simulink model "OMSv1_1_SSI"  (Simulink 6.5)
settings: Solver=ode4  SolverMode=SingleTasking  StartTime=0.0  StopTime=2.5  FixedStep=0.001  MaxStep=0.001  RelTol=1e-3  AbsTol=1e-3
undefined symbols (not defined in the file): alexlaw, bs_onoff, bs_scale, bsfsacrit, bsfsvcrit, cnsgain, fs_onoff, fs_scale, fsdelaycalc, ltdrk, phasicgain, pmcgain, pmctau2, pmctau3, saccrefract, saccsw, spgain, tonicgain, tvrD, tvrN, velnoise, velreconsw
(part 5 of 8)

== system OMSv1_1_SSI/OMSv1.1_SSI 01/27/03/IM CN-LMLN/Saccade Enable/Enable Contol/2 ms ==
  note: init Q = 0
  note: Stretch the duration of an input pulse, latching it at its value at pulse onset.
  note: The one integration step delay before the S&H block's S/H (bottom) input insures
      | that the input value to be latched is available to theS&H block's top input
      | before the S&H block tries to 'hold'.
  note: The start of the input pulse causes the value on input 1 to be held starting when the leading
      | edge occurs, and this value remains latched until 'delay' seconds after the pulse ends (trailing edge).
  note: 11/22/99
  note: init = 0
  note: init = 0
  value(in) : Inport
  " x/1000" : Constant  Orientation=up  Value=0.001
  Latch1 : Subsystem  mask(Latch){@1=0}
      mask prompts: @1 "Initial State for Output "Q":"
      mask help: Latch
      mask init:
      | ini=(@1~=0);
      mask Help: Latches the S input.  When S (set) is one, the Q output  becomes one.  The output remains one until the R (reset) input becomes one, forcing the output to zero.  If both R and S are one, the latch will be in an undefined state.
      mask Display: disp('S   Q\n\nR  !Q')
  Product : Product  SaturateOnIntegerOverflow=on  RndMeth=Zero  InputSameDT=on
  SampHold?2 : Subsystem
      mask Display: disp('S=L\nH=H')
  Variable Transport Delay : VariableTransportDelay  MaximumDelay=10
  leading edge detect : Subsystem
      mask Display: disp('Leading\nEdge Det')
  loop breaker2 : Memory
  stretch : Constant  Value=prolong
  trailing edge detect : Subsystem
      mask Display: disp('Trailing\nEdge Det')
  value(out) : Outport  InitialOutput=0
  wires:
  value(in)/1 -> leading edge detect/1(in_1), trailing edge detect/1(in_1), SampHold?2/1(Input)
  Variable Transport Delay/1 -> Latch1/2(in_2)
  trailing edge detect/1(out_1) -> Variable Transport Delay/1
  leading edge detect/1(out_1) -> Latch1/1(in_1)
  Latch1/1(out_1) -> loop breaker2/1
  SampHold?2/1(output) -> value(out)/1
  loop breaker2/1 -> SampHold?2/2(S/H?)
  stretch/1 -> Product/1
  Product/1 -> Variable Transport Delay/2
  " x/1000"/1 -> Product/2

== system OMSv1_1_SSI/OMSv1.1_SSI 01/27/03/IM CN-LMLN/Saccade Enable/Enable Contol/50 ms ==
  note: init = 0
  note: init = 0
  note: 11/22/99
  note: The start of the input pulse causes the value on input 1 to be held starting when the leading
      | edge occurs, and this value remains latched until 'delay' seconds after the pulse ends (trailing edge).
  note: The one integration step delay before the S&H block's S/H (bottom) input insures
      | that the input value to be latched is available to theS&H block's top input
      | before the S&H block tries to 'hold'.
  note: Stretch the duration of an input pulse, latching it at its value at pulse onset.
  note: init Q = 0
  value(in) : Inport
  " x/1000" : Constant  Orientation=up  Value=0.001
  Latch1 : Subsystem  mask(Latch){@1=0}
      mask prompts: @1 "Initial State for Output "Q":"
      mask help: Latch
      mask init:
      | ini=(@1~=0);
      mask Help: Latches the S input.  When S (set) is one, the Q output  becomes one.  The output remains one until the R (reset) input becomes one, forcing the output to zero.  If both R and S are one, the latch will be in an undefined state.
      mask Display: disp('S   Q\n\nR  !Q')
  Product : Product  SaturateOnIntegerOverflow=on  RndMeth=Zero  InputSameDT=on
  SampHold?2 : Subsystem
      mask Display: disp('S=L\nH=H')
  Variable Transport Delay : VariableTransportDelay  MaximumDelay=10
  leading edge detect : Subsystem
      mask Display: disp('Leading\nEdge Det')
  loop breaker2 : Memory
  stretch : Constant  Value=prolong
  trailing edge detect : Subsystem
      mask Display: disp('Trailing\nEdge Det')
  value(out) : Outport  InitialOutput=0
  wires:
  " x/1000"/1 -> Product/2
  Product/1 -> Variable Transport Delay/2
  stretch/1 -> Product/1
  loop breaker2/1 -> SampHold?2/2(S/H?)
  SampHold?2/1(output) -> value(out)/1
  Latch1/1(out_1) -> loop breaker2/1
  leading edge detect/1(out_1) -> Latch1/1(in_1)
  trailing edge detect/1(out_1) -> Variable Transport Delay/1
  Variable Transport Delay/1 -> Latch1/2(in_2)
  value(in)/1 -> SampHold?2/1(Input), trailing edge detect/1(in_1), leading edge detect/1(in_1)

== system OMSv1_1_SSI/OMSv1.1_SSI 01/27/03/IM CN-LMLN/Saccade Enable/Enable Contol/Boolify ==
  In1 : Inport
  Abs2 : Abs  SaturateOnIntegerOverflow=on
  direction1 : Subsystem
      mask Type: Sign
      mask Description: y = sign(x)
      mask Help: Sign Function:\n\t\t\ty = 1 if x > 0\n\t\t\ty = 0 if x = 0\n\t\t\ty = -1 if x < 0
      mask Display: plot(-50,-50,50,50,[-50,50],[0,0],[0,0],[-50,50],[-40,0],[-30,-30],[0,40],[30,30])
  Out1 : Outport  InitialOutput=0
  wires:
  Abs2/1 -> direction1/1(in_1)
  In1/1 -> Abs2/1
  direction1/1(out_1) -> Out1/1

== system OMSv1_1_SSI/OMSv1.1_SSI 01/27/03/IM CN-LMLN/Saccade Enable/Enable Contol/Boolify1 ==
  In1 : Inport
  Abs2 : Abs  SaturateOnIntegerOverflow=on
  direction1 : Subsystem
      mask Type: Sign
      mask Description: y = sign(x)
      mask Help: Sign Function:\n\t\t\ty = 1 if x > 0\n\t\t\ty = 0 if x = 0\n\t\t\ty = -1 if x < 0
      mask Display: plot(-50,-50,50,50,[-50,50],[0,0],[0,0],[-50,50],[-40,0],[-30,-30],[0,40],[30,30])
  Out1 : Outport  InitialOutput=0
  wires:
  Abs2/1 -> direction1/1(in_1)
  In1/1 -> Abs2/1
  direction1/1(out_1) -> Out1/1

== system OMSv1_1_SSI/OMSv1.1_SSI 01/27/03/IM CN-LMLN/Saccade Enable/Enable Contol/Boolify2 ==
  In1 : Inport
  Abs2 : Abs  SaturateOnIntegerOverflow=on
  direction1 : Subsystem
      mask Type: Sign
      mask Description: y = sign(x)
      mask Help: Sign Function:\n\t\t\ty = 1 if x > 0\n\t\t\ty = 0 if x = 0\n\t\t\ty = -1 if x < 0
      mask Display: plot(-50,-50,50,50,[-50,50],[0,0],[0,0],[-50,50],[-40,0],[-30,-30],[0,40],[30,30])
  Out1 : Outport  InitialOutput=0
  wires:
  Abs2/1 -> direction1/1(in_1)
  In1/1 -> Abs2/1
  direction1/1(out_1) -> Out1/1

== system OMSv1_1_SSI/OMSv1.1_SSI 01/27/03/IM CN-LMLN/Saccade Enable/Enable Contol/ECPY Timing ==
  note: ECPY Timing
  note: (Init input:0)
  note: (Init input: 1)
  note: (FF init state: Q=0)
  note: (Init input: 0)
  note: (FF init state: Q=0)
  note: (((see original refract latch block for full description of operation.)))
  note: This signal is used by the Internal Monitor to decide when to compare EFERENCE COPY eye position with old eye position to decide if an appropriate saccade was made.
  note: This block outputs an ENABLE signal xx milliseconds long (set in "enable duration"), starting xx milliseconds (set in "post-pulse delay time") AFTER the input pulse concludes.
  note: If the FF init state is 0, then the block's initial output will be zero. If the FF init state is 1, then the block's initial output will be one.
  note: Corrective Saccades
  ECPY EnCntr [ecenctrl] : Inport
  Latch2 : Subsystem  mask(Latch){@1=0}
      mask prompts: @1 "Initial State for Output "Q":"
      mask help: Latch
      mask init:
      | ini=(@1~=0);
      mask Help: Latches the S input.  When S (set) is one, the Q output becomes one.  The output remains one until the R (reset) input becomes one, forcing the output to zero.  If both R and S are one, the latch will be in an undefined state.
      mask Display: disp('S   Q\n\nR  !Q')
  Latch4 : Subsystem  mask(Latch){@1=0}
      mask prompts: @1 "Initial State for Output "Q":"
      mask help: Latch
      mask init:
      | ini=(@1~=0);
      mask Help: Latches the S input.  When S (set) is one, the Q output becomes one.  The output remains one until the R (reset) input becomes one, forcing the output to zero.  If both R and S are one, the latch will be in an undefined state.
      mask Display: disp('S   Q\n\nR  !Q')
  Switch1 : Switch  Threshold=.5  SaturateOnIntegerOverflow=on  InputSameDT=on
  Threshold 3 : Constant  Orientation=left  Value=0
  enab dur 10ms : TransportDelay  DelayTime=.01  InitialOutput=1
  leading edge detect : Subsystem
      mask Display: disp('Leading\nEdge Det')
  leading edge detect1 : Subsystem
      mask Display: disp('Leading\nEdge Det')
  loop breaker : Memory  Orientation=left
  or : Logic  Operator=OR
  post-pulse delay 130ms : TransportDelay  DelayTime=.13
  trailing edge detect : Subsystem
      mask Display: disp('Trailing\nEdge Det')
  ECPY Enable [ecpyenab] : Outport  InitialOutput=0
  wires:
  or/1 -> Latch4/2(in_2)
  trailing edge detect/1(out_1) -> or/1, post-pulse delay 130ms/1
  Switch1/1 -> leading edge detect1/1(in_1), trailing edge detect/1(in_1)
  leading edge detect1/1(out_1) -> or/2
  ECPY EnCntr [ecenctrl]/1 -> Switch1/1
  Threshold 3/1 -> Switch1/3
  loop breaker/1 -> Switch1/2
  Latch2/1(out_1) -> ECPY Enable [ecpyenab]/1
  leading edge detect/1(out_1) -> enab dur 10ms/1, Latch2/1(in_1)
  enab dur 10ms/1 -> Latch2/2(in_2)
  Latch2/2(out_2) -> loop breaker/1
  post-pulse delay 130ms/1 -> Latch4/1(in_1)
  Latch4/1(out_1) -> leading edge detect/1(in_1)

== system OMSv1_1_SSI/OMSv1.1_SSI 01/27/03/IM CN-LMLN/Saccade Enable/Enable Contol/Latch1 ==
  in_1 : Inport
  in_2 : Inport  Port=2
  Demux : Demux  Outputs=2
  Logic : CombinatorialLogic  TruthTable=[0 1;0 1;1 0;0 1;1 0;0 1;1 0;1 0]
  Memory : Memory  Orientation=left  X0=ini
  Mux : Mux  Inputs=3
  out_1 : Outport  InitialOutput=0
  out_2 : Outport  Port=2  InitialOutput=0
  wires:
  Demux/2 -> out_2/1
  Logic/1 -> Demux/1
  Mux/1 -> Logic/1
  Demux/1 -> out_1/1, Memory/1
  Memory/1 -> Mux/1
  in_1/1 -> Mux/2
  in_2/1 -> Mux/3

== system OMSv1_1_SSI/OMSv1.1_SSI 01/27/03/IM CN-LMLN/Saccade Enable/Enable Contol/Latch2 ==
  in_1 : Inport
  in_2 : Inport  Port=2
  Demux : Demux  Outputs=2
  Logic : CombinatorialLogic  TruthTable=[0 1;0 1;1 0;0 1;1 0;0 1;1 0;1 0]
  Memory : Memory  Orientation=left  X0=ini
  Mux : Mux  Inputs=3
  out_1 : Outport  InitialOutput=0
  out_2 : Outport  Port=2  InitialOutput=0
  wires:
  in_2/1 -> Mux/3
  in_1/1 -> Mux/2
  Memory/1 -> Mux/1
  Demux/1 -> Memory/1, out_1/1
  Mux/1 -> Logic/1
  Logic/1 -> Demux/1
  Demux/2 -> out_2/1

== system OMSv1_1_SSI/OMSv1.1_SSI 01/27/03/IM CN-LMLN/Saccade Enable/Enable Contol/Latch3 ==
  in_1 : Inport
  in_2 : Inport  Port=2
  Demux : Demux  Outputs=2
  Logic : CombinatorialLogic  TruthTable=[0 1;0 1;1 0;0 1;1 0;0 1;1 0;1 0]
  Memory : Memory  Orientation=left  X0=ini
  Mux : Mux  Inputs=3
  out_1 : Outport  InitialOutput=0
  out_2 : Outport  Port=2  InitialOutput=0
  wires:
  Demux/2 -> out_2/1
  Logic/1 -> Demux/1
  Mux/1 -> Logic/1
  Demux/1 -> out_1/1, Memory/1
  Memory/1 -> Mux/1
  in_1/1 -> Mux/2
  in_2/1 -> Mux/3

== system OMSv1_1_SSI/OMSv1.1_SSI 01/27/03/IM CN-LMLN/Saccade Enable/Enable Contol/event timer1 ==
  note: Resettable
      | Event Timer
  note: This block is an RESETTABLE EVENT TIMER.  It outputs a spike of unit height xx milliseconds
      | (set by "timer value") after it detects an event ( i.e a TRAILING edge which represents the end of a
      |  saccadic pulse)
  note: (Init input: 0)
  note: (FF init state: Q=0)
  note: (Init input: 0)
  note: Therefore, an event first RESETS and then SETS the flip-flop.
  note: The "OR" gate allows either of these conditions to reset the circuit.  The delay before the
      | "S" input of the flip-flop prevents both "S" and "R" from being set simultaneously, because
      | this would put the flip-flop in an undefined state.
  note: The real trick here is understanding how to reload the countdown.
      | It resets if either of two conditions is met:
  note: It has TWO modes: 1) Event resettable and 2) Event Non-resettable
  note: In 1), Any event (leading or trailing edge) will reset the counter so that it
      | counts down from the end trailing edge) of that event.
  note: 1) The count reaches its limit (set in "timer value") -- Both case 1) and 2)
  note: 2) A new event (leading or trailing edge) is detected. -- Only case 1)
  note: In 2) Subsequent events DO NOT reset the counter; it only resets when it
      | reaches zero
  SW out : Inport
  _timer value (port) : Inport  Port=2
  1 msec : TransportDelay  DelayTime=.001
  Clock : Clock
      settings: Decimation=10
  Latch1 : Subsystem  mask(Latch){@1=0}
      mask prompts: @1 "Initial State for Output "Q":"
      mask help: Latch
      mask init:
      | ini=(@1~=0);
      mask Help: Latches the S input.  When S (set) is one, the Q output  becomes one.  The output remains one until the R (reset) input becomes one, forcing the output to zero.  If both R and S are one, the latch will be in an undefined state.
      mask Display: disp('S   Q\n\nR  !Q')
  Logical Operator : Logic  Operator=OR  Inputs=3
  Logical Operator1 : Logic
  Logical Operator2 : Logic
  Relational Operator : RelationalOperator  InputSameDT=on
  SampHold?1 : Subsystem
      mask Display: disp('S&H\n(S=L)\n(H=H)')
  Sum : Sum  Inputs=+-  SaturateOnIntegerOverflow=on  InputSameDT=on
  event resettable? : Constant  Orientation=up
  leading edge detect : Subsystem
      mask Display: disp('Leading\nEdge Det')
  loop breaker : Memory  Orientation=left
  trailing edge detect : Subsystem
      mask Display: disp('Trailing\nEdge Det')
  FF Reset : Outport  InitialOutput=0
  wires:
  _timer value (port)/1 -> Relational Operator/2
  1 msec/1 -> Latch1/1(in_1)
  Logical Operator/1 -> Latch1/2(in_2)
  SampHold?1/1(output) -> Sum/2
  Relational Operator/1 -> loop breaker/1, FF Reset/1
  SW out/1 -> trailing edge detect/1(in_1), leading edge detect/1(in_1)
  Clock/1 -> Sum/1, SampHold?1/1(Input)
  Sum/1 -> Relational Operator/1
  Latch1/1(out_1) -> SampHold?1/2(S/H?)
  loop breaker/1 -> Logical Operator/3
  Logical Operator1/1 -> Logical Operator/1
  trailing edge detect/1(out_1) -> Logical Operator1/1, 1 msec/1
  Logical Operator2/1 -> Logical Operator/2
  leading edge detect/1(out_1) -> Logical Operator2/1
  event resettable?/1 -> Logical Operator2/2, Logical Operator1/2

== system OMSv1_1_SSI/OMSv1.1_SSI 01/27/03/IM CN-LMLN/Saccade Enable/Enable Contol/leading edge detect ==
  note: It is also possible to remove the SIGNUM function
      | and the '==', and replace them with a simple
      | switch with a threshold of (say) 150 or so.
  note: leading edge detection
  in_1 : Inport
  Abs : Abs  SaturateOnIntegerOverflow=on
  Derivative : Derivative
  Relational Operator : RelationalOperator  Operator===  InputSameDT=on
  Sign : Subsystem
      mask Type: Sign
      mask Description: y = sign(x)
      mask Help: Sign Function:\n\t\t\ty = 1 if x > 0\n\t\t\ty = 0 if x = 0\n\t\t\ty = -1 if x < 0
      mask Display: plot(-50,-50,50,50,[-50,50],[0,0],[0,0],[-50,50],[-40,0],[-30,-30],[0,40],[30,30])
  Threshold 1 : Constant
  out_1 : Outport  InitialOutput=0
  wires:
  Abs/1 -> Derivative/1
  Derivative/1 -> Sign/1(in_1)
  Sign/1(out_1) -> Relational Operator/1
  Threshold 1/1 -> Relational Operator/2
  Relational Operator/1 -> out_1/1
  in_1/1 -> Abs/1

== system OMSv1_1_SSI/OMSv1.1_SSI 01/27/03/IM CN-LMLN/Saccade Enable/Enable Contol/leading edge detect2 ==
  note: leading edge detection
  note: It is also possible to remove the SIGNUM function
      | and the '==', and replace them with a simple
      | switch with a threshold of (say) 150 or so.
  in_1 : Inport
  Abs : Abs  SaturateOnIntegerOverflow=on
  Derivative : Derivative
  Relational Operator : RelationalOperator  Operator===  InputSameDT=on
  Sign : Subsystem
      mask Type: Sign
      mask Description: y = sign(x)
      mask Help: Sign Function:\n\t\t\ty = 1 if x > 0\n\t\t\ty = 0 if x = 0\n\t\t\ty = -1 if x < 0
      mask Display: plot(-50,-50,50,50,[-50,50],[0,0],[0,0],[-50,50],[-40,0],[-30,-30],[0,40],[30,30])
  Threshold 1 : Constant
  out_1 : Outport  InitialOutput=0
  wires:
  in_1/1 -> Abs/1
  Relational Operator/1 -> out_1/1
  Threshold 1/1 -> Relational Operator/2
  Sign/1(out_1) -> Relational Operator/1
  Derivative/1 -> Sign/1(in_1)
  Abs/1 -> Derivative/1

== system OMSv1_1_SSI/OMSv1.1_SSI 01/27/03/IM CN-LMLN/Saccade Enable/Enable Contol/trailing edge detect ==
  note: It is also possible to remove the SIGNUM function
      | and the '==', and replace them with a simple
      | switch with a threshold of (say) 150 or so.
  note: trailing edge detection
  PG : Inport
  Abs : Abs  SaturateOnIntegerOverflow=on
  Derivative : Derivative
  Relational Operator : RelationalOperator  Operator===  InputSameDT=on
  Sign : Subsystem
      mask Type: Sign
      mask Description: y = sign(x)
      mask Help: Sign Function:\n\t\t\ty = 1 if x > 0\n\t\t\ty = 0 if x = 0\n\t\t\ty = -1 if x < 0
      mask Display: plot(-50,-50,50,50,[-50,50],[0,0],[0,0],[-50,50],[-40,0],[-30,-30],[0,40],[30,30])
  Threshold 1 : Constant  Value=-1
  Latch R : Outport  InitialOutput=0
  wires:
  Abs/1 -> Derivative/1
  Derivative/1 -> Sign/1(in_1)
  Sign/1(out_1) -> Relational Operator/1
  Threshold 1/1 -> Relational Operator/2
  Relational Operator/1 -> Latch R/1
  PG/1 -> Abs/1

== system OMSv1_1_SSI/OMSv1.1_SSI 01/27/03/IM CN-LMLN/Saccade Enable/LN FPh Gen/DZ 4 ==
  note: This block is a better implementation of a dead zone than  the
      | block supplied by SIMULINK, because here we don't _subtract_
      | the dead zone from the rest of output.
  note: We just output zero when the dead zone is in effect, and leave the
      |  output alone the rest of the time.
  in_1 : Inport
  Abs : Abs  Orientation=down  SaturateOnIntegerOverflow=on
  Relational Operator : RelationalOperator  InputSameDT=on
  Switch6 : Switch  Threshold=.5  SaturateOnIntegerOverflow=on  InputSameDT=on
  dead zone : Constant  Orientation=up  Value=4
  pos (deg) criterion1 : Constant  Orientation=left  Value=0
  out_1 : Outport  InitialOutput=0
  wires:
  Switch6/1 -> out_1/1
  in_1/1 -> Switch6/1, Abs/1
  Abs/1 -> Relational Operator/1
  pos (deg) criterion1/1 -> Switch6/3
  dead zone/1 -> Relational Operator/2
  Relational Operator/1 -> Switch6/2

== system OMSv1_1_SSI/OMSv1.1_SSI 01/27/03/IM CN-LMLN/Saccade Enable/LN FPh Gen/Latch1 ==
  in_1 : Inport
  in_2 : Inport  Port=2
  Demux : Demux  Outputs=2
  Logic : CombinatorialLogic  TruthTable=[0 1;0 1;1 0;0 1;1 0;0 1;1 0;1 0]
  Memory : Memory  Orientation=left  X0=ini
  Mux : Mux  Inputs=3
  out_1 : Outport  InitialOutput=0
  out_2 : Outport  Port=2  InitialOutput=0
  wires:
  in_2/1 -> Mux/3
  in_1/1 -> Mux/2
  Memory/1 -> Mux/1
  Demux/1 -> Memory/1, out_1/1
  Mux/1 -> Logic/1
  Logic/1 -> Demux/1
  Demux/2 -> out_2/1

== system OMSv1_1_SSI/OMSv1.1_SSI 01/27/03/IM CN-LMLN/Saccade Enable/LN FPh Gen/SampHold?1 ==
  note: When "S/H?" is HIGH, then "Input" is switched directly to the
      | output ("sample").  When "S/H?" is LOW, the current output is
      | maintained ("hold").
  Input : Inport
  S/H? : Inport  Port=2
  Memory : Memory  Orientation=left
  Sign : Subsystem
      mask Type: Sign
      mask Description: y = sign(x)
      mask Help: Sign Function:\n\t\t\ty = 1 if x > 0\n\t\t\ty = 0 if x = 0\n\t\t\ty = -1 if x < 0
      mask Display: plot(-50,-50,50,50,[-50,50],[0,0],[0,0],[-50,50],[-40,0],[-30,-30],[0,40],[30,30])
  Switch2 : Switch  Threshold=0.5  SaturateOnIntegerOverflow=on  InputSameDT=on
  output : Outport  InitialOutput=0
  wires:
  Memory/1 -> Switch2/3
  Input/1 -> Switch2/1
  Switch2/1 -> Memory/1, output/1
  Sign/1(out_1) -> Switch2/2
  S/H?/1 -> Sign/1(in_1)

== system OMSv1_1_SSI/OMSv1.1_SSI 01/27/03/IM CN-LMLN/Saccade Enable/LN FPh Gen/event timer1 ==
  note: Resettable
      | Event Timer
  note: This block is an RESETTABLE EVENT TIMER.  It outputs a spike of unit height xx milliseconds
      | (set by "timer value") after it detects an event ( i.e a TRAILING edge which represents the end of a
      |  saccadic pulse)
  note: (Init input: 0)
  note: (FF init state: Q=0)
  note: (Init input: 0)
  note: Therefore, an event first RESETS and then SETS the flip-flop.
  note: The "OR" gate allows either of these conditions to reset the circuit.  The delay before the
      | "S" input of the flip-flop prevents both "S" and "R" from being set simultaneously, because
      | this would put the flip-flop in an undefined state.
  note: The real trick here is understanding how to reload the countdown.
      | It resets if either of two conditions is met:
  note: It has TWO modes: 1) Event resettable and 2) Event Non-resettable
  note: In 1), Any event (leading or trailing edge) will reset the counter so that it
      | counts down from the end trailing edge) of that event.
  note: 1) The count reaches its limit (set in "timer value") -- Both case 1) and 2)
  note: 2) A new event (leading or trailing edge) is detected. -- Only case 1)
  note: In 2) Subsequent events DO NOT reset the counter; it only resets when it
      | reaches zero
  _PG : Inport
  _timer value (port) : Inport  Port=2
  1 msec : TransportDelay  DelayTime=.001
  Clock : Clock
      settings: Decimation=10
  Latch1 : Subsystem  mask(Latch){@1=0}
      mask prompts: @1 "Initial State for Output "Q":"
      mask help: Latch
      mask init:
      | ini=(@1~=0);
      mask Help: Latches the S input.  When S (set) is one, the Q output  becomes one.  The output remains one until the R (reset) input becomes one, forcing the output to zero.  If both R and S are one, the latch will be in an undefined state.
      mask Display: disp('S   Q\n\nR  !Q')
  Logical Operator : Logic  Operator=OR  Inputs=3
  Logical Operator1 : Logic
  Logical Operator2 : Logic
  Relational Operator : RelationalOperator  InputSameDT=on
  SampHold?1 : Subsystem
      mask Display: disp('S&H\n(S=L)\n(H=H)')
  Sum : Sum  Inputs=+-  SaturateOnIntegerOverflow=on  InputSameDT=on
  event resettable? : Constant  Orientation=up
  leading edge detect : Subsystem
      mask Display: disp('Leading\nEdge Det')
  loop breaker : Memory  Orientation=left
  trailing edge detect : Subsystem
      mask Display: disp('Trailing\nEdge Det')
  out_1 : Outport  InitialOutput=0
  wires:
  _timer value (port)/1 -> Relational Operator/2
  1 msec/1 -> Latch1/1(in_1)
  Logical Operator/1 -> Latch1/2(in_2)
  SampHold?1/1(output) -> Sum/2
  Relational Operator/1 -> loop breaker/1, out_1/1
  _PG/1 -> trailing edge detect/1(in_1), leading edge detect/1(in_1)
  Clock/1 -> Sum/1, SampHold?1/1(Input)
  Sum/1 -> Relational Operator/1
  Latch1/1(out_1) -> SampHold?1/2(S/H?)
  loop breaker/1 -> Logical Operator/3
  Logical Operator1/1 -> Logical Operator/1
  trailing edge detect/1(out_1) -> Logical Operator1/1, 1 msec/1
  Logical Operator2/1 -> Logical Operator/2
  leading edge detect/1(out_1) -> Logical Operator2/1
  event resettable?/1 -> Logical Operator2/2, Logical Operator1/2

== system OMSv1_1_SSI/OMSv1.1_SSI 01/27/03/IM CN-LMLN/Saccade Enable/LN FPh Gen/leading edge detect ==
  note: leading edge detection
  in_1 : Inport
  Abs : Abs  SaturateOnIntegerOverflow=on
  Derivative : Derivative
  Relational Operator : RelationalOperator  Operator===  InputSameDT=on
  Sign : Subsystem
      mask Type: Sign
      mask Description: y = sign(x)
      mask Help: Sign Function:\n\t\t\ty = 1 if x > 0\n\t\t\ty = 0 if x = 0\n\t\t\ty = -1 if x < 0
      mask Display: plot(-50,-50,50,50,[-50,50],[0,0],[0,0],[-50,50],[-40,0],[-30,-30],[0,40],[30,30])
  Threshold 1 : Constant
  out_1 : Outport  InitialOutput=0
  wires:
  in_1/1 -> Abs/1
  Relational Operator/1 -> out_1/1
  Threshold 1/1 -> Relational Operator/2
  Sign/1(out_1) -> Relational Operator/1
  Derivative/1 -> Sign/1(in_1)
  Abs/1 -> Derivative/1

== system OMSv1_1_SSI/OMSv1.1_SSI 01/27/03/IM CN-LMLN/Saccade Enable/Ret FB sample/Boolify ==
  In1 : Inport
  Abs2 : Abs  SaturateOnIntegerOverflow=on
  direction1 : Subsystem
      mask Type: Sign
      mask Description: y = sign(x)
      mask Help: Sign Function:\n\t\t\ty = 1 if x > 0\n\t\t\ty = 0 if x = 0\n\t\t\ty = -1 if x < 0
      mask Display: plot(-50,-50,50,50,[-50,50],[0,0],[0,0],[-50,50],[-40,0],[-30,-30],[0,40],[30,30])
  Out1 : Outport  InitialOutput=0
  wires:
  Abs2/1 -> direction1/1(in_1)
  In1/1 -> Abs2/1
  direction1/1(out_1) -> Out1/1

== system OMSv1_1_SSI/OMSv1.1_SSI 01/27/03/IM CN-LMLN/Saccade Enable/Ret FB sample/Boolify1 ==
  In1 : Inport
  Abs2 : Abs  SaturateOnIntegerOverflow=on
  direction1 : Subsystem
      mask Type: Sign
      mask Description: y = sign(x)
      mask Help: Sign Function:\n\t\t\ty = 1 if x > 0\n\t\t\ty = 0 if x = 0\n\t\t\ty = -1 if x < 0
      mask Display: plot(-50,-50,50,50,[-50,50],[0,0],[0,0],[-50,50],[-40,0],[-30,-30],[0,40],[30,30])
  Out1 : Outport  InitialOutput=0
  wires:
  Abs2/1 -> direction1/1(in_1)
  In1/1 -> Abs2/1
  direction1/1(out_1) -> Out1/1

== system OMSv1_1_SSI/OMSv1.1_SSI 01/27/03/IM CN-LMLN/Saccade Enable/Ret FB sample/Latch1 ==
  in_1 : Inport
  in_2 : Inport  Port=2
  Demux : Demux  Outputs=2
  Logic : CombinatorialLogic  TruthTable=[0 1;0 1;1 0;0 1;1 0;0 1;1 0;1 0]
  Memory : Memory  Orientation=left  X0=ini
  Mux : Mux  Inputs=3
  out_1 : Outport  InitialOutput=0
  out_2 : Outport  Port=2  InitialOutput=0
  wires:
  Demux/2 -> out_2/1
  Logic/1 -> Demux/1
  Mux/1 -> Logic/1
  Demux/1 -> out_1/1, Memory/1
  Memory/1 -> Mux/1
  in_1/1 -> Mux/2
  in_2/1 -> Mux/3

== system OMSv1_1_SSI/OMSv1.1_SSI 01/27/03/IM CN-LMLN/Saccade Enable/Ret FB sample/Latch2 ==
  in_1 : Inport
  in_2 : Inport  Port=2
  Demux : Demux  Outputs=2
  Logic : CombinatorialLogic  TruthTable=[0 1;0 1;1 0;0 1;1 0;0 1;1 0;1 0]
  Memory : Memory  Orientation=left  X0=ini
  Mux : Mux  Inputs=3
  out_1 : Outport  InitialOutput=0
  out_2 : Outport  Port=2  InitialOutput=0
  wires:
  in_2/1 -> Mux/3
  in_1/1 -> Mux/2
  Memory/1 -> Mux/1
  Demux/1 -> out_1/1, Memory/1
  Mux/1 -> Logic/1
  Logic/1 -> Demux/1
  Demux/2 -> out_2/1

== system OMSv1_1_SSI/OMSv1.1_SSI 01/27/03/IM CN-LMLN/Saccade Enable/Ret FB sample/Sign ==
  in_1 : Inport
  Constant : Constant  Value=0
  Relational Operator : RelationalOperator  Operator=>  InputSameDT=on
  Relational Operator1 : RelationalOperator  Operator=<  InputSameDT=on
  Sum : Sum  Inputs=+-  SaturateOnIntegerOverflow=on  InputSameDT=on
  out_1 : Outport  InitialOutput=0
  wires:
  in_1/1 -> Relational Operator/1, Relational Operator1/1
  Constant/1 -> Relational Operator1/2, Relational Operator/2
  Relational Operator1/1 -> Sum/2
  Relational Operator/1 -> Sum/1
  Sum/1 -> out_1/1

== system OMSv1_1_SSI/OMSv1.1_SSI 01/27/03/IM CN-LMLN/Saccade Enable/Ret FB sample/event timer2 ==
  note: Resettable
      | Event Timer
  note: (Init input: 0)
  note: (FF init state: Q=0)
  note: (Init input: 0)
  note: In 2) Subsequent events DO NOT reset the counter; it only resets when it
      | reaches zero
  note: 2) A new event (leading or trailing edge) is detected. -- Only case 1)
  note: 1) The count reaches its limit (set in "timer value") -- Both case 1) and 2)
  note: In 1), A leading or trailing edge will reset the counter so that it
      | counts down from the end trailing edge) of that event.
  note: It has TWO modes: 1) Event resettable and 2) Event Non-resettable
  note: The real trick here is understanding how to reload the countdown.
      | It resets if either of two conditions is met:
  note: The "OR" gate allows either of these conditions to reset the circuit.  The delay before the
      | "S" input of the flip-flop prevents both "S" and "R" from being set simultaneously, because
      | this would put the flip-flop in an undefined state.
  note: Therefore, an event first RESETS and then SETS the flip-flop.
  note: This block is an RESETTABLE EVENT TIMER.  It outputs a spike of unit height xx milliseconds
      | (set by "timer value") after it detects an event ( i.e a TRAILING edge which represents the end of a
      |  saccadic pulse)
  RetFB EnCntrl : Inport
  _timer value (port) : Inport  Port=2
  1 msec : TransportDelay  DelayTime=.001
  Clock : Clock
      settings: Decimation=10
  Latch1 : Subsystem  mask(Latch){@1=0}
      mask prompts: @1 "Initial State for Output "Q":"
      mask help: Latch
      mask init:
      | ini=(@1~=0);
      mask Help: Latches the S input.  When S (set) is one, the Q output  becomes one.  The output remains one until the R (reset) input becomes one, forcing the output to zero.  If both R and S are one, the latch will be in an undefined state.
      mask Display: disp('S   Q\n\nR  !Q')
  Logical Operator : Logic  Operator=OR  Inputs=3
  Logical Operator1 : Logic
  Logical Operator2 : Logic
  Relational Operator : RelationalOperator  InputSameDT=on
  SampHold?1 : Subsystem
      mask Display: disp('S&H\n(S=L)\n(H=H)')
  Sum : Sum  Inputs=+-  SaturateOnIntegerOverflow=on  InputSameDT=on
  event resettable? : Constant  Orientation=up
  leading edge detect : Subsystem
      mask Display: disp('Leading\nEdge Det')
  loop breaker : Memory  Orientation=left
  trailing edge detect : Subsystem
      mask Display: disp('Trailing\nEdge Det')
  outFF : Outport  InitialOutput=0
  wires:
  RetFB EnCntrl/1 -> trailing edge detect/1(in_1), leading edge detect/1(in_1)
  event resettable?/1 -> Logical Operator1/2, Logical Operator2/2
  leading edge detect/1(out_1) -> Logical Operator2/1
  Logical Operator2/1 -> Logical Operator/2
  trailing edge detect/1(out_1) -> 1 msec/1, Logical Operator1/1
  Logical Operator1/1 -> Logical Operator/1
  loop breaker/1 -> Logical Operator/3
  Latch1/1(out_1) -> SampHold?1/2(S/H?)
  Sum/1 -> Relational Operator/1
  Clock/1 -> SampHold?1/1(Input), Sum/1
  Relational Operator/1 -> outFF/1, loop breaker/1
  SampHold?1/1(output) -> Sum/2
  Logical Operator/1 -> Latch1/2(in_2)
  1 msec/1 -> Latch1/1(in_1)
  _timer value (port)/1 -> Relational Operator/2

== system OMSv1_1_SSI/OMSv1.1_SSI 01/27/03/IM CN-LMLN/Saccade Enable/Ret FB sample/event timer3 ==
  note: This block is an RESETTABLE EVENT TIMER.  It outputs a spike of unit height xx milliseconds
      | (set by "timer value") after it detects an event ( i.e a TRAILING edge which represents the end of a
      |  saccadic pulse)
  note: Therefore, an event first RESETS and then SETS the flip-flop.
  note: The "OR" gate allows either of these conditions to reset the circuit.  The delay before the
      | "S" input of the flip-flop prevents both "S" and "R" from being set simultaneously, because
      | this would put the flip-flop in an undefined state.
  note: The real trick here is understanding how to reload the countdown.
      | It resets if either of two conditions is met:
  note: It has TWO modes: 1) Event resettable and 2) Event Non-resettable
  note: In 1), A leading or trailing edge will reset the counter so that it
      | counts down from the end trailing edge) of that event.
  note: 1) The count reaches its limit (set in "timer value") -- Both case 1) and 2)
  note: 2) A new event (leading or trailing edge) is detected. -- Only case 1)
  note: In 2) Subsequent events DO NOT reset the counter; it only resets when it
      | reaches zero
  note: (Init input: 0)
  note: (FF init state: Q=0)
  note: (Init input: 0)
  note: Resettable
      | Event Timer
  RetFB EnCntrl : Inport
  _timer value (port) : Inport  Port=2
  1 msec : TransportDelay  DelayTime=.001
  Clock : Clock
      settings: Decimation=10
  Latch1 : Subsystem  mask(Latch){@1=0}
      mask prompts: @1 "Initial State for Output "Q":"
      mask help: Latch
      mask init:
      | ini=(@1~=0);
      mask Help: Latches the S input.  When S (set) is one, the Q output  becomes one.  The output remains one until the R (reset) input becomes one, forcing the output to zero.  If both R and S are one, the latch will be in an undefined state.
      mask Display: disp('S   Q\n\nR  !Q')
  Logical Operator : Logic  Operator=OR  Inputs=3
  Logical Operator1 : Logic
  Logical Operator2 : Logic
  Relational Operator : RelationalOperator  InputSameDT=on
  SampHold?1 : Subsystem
      mask Display: disp('S&H\n(S=L)\n(H=H)')
  Sum : Sum  Inputs=+-  SaturateOnIntegerOverflow=on  InputSameDT=on
  event resettable? : Constant  Orientation=up
  leading edge detect : Subsystem
      mask Display: disp('Leading\nEdge Det')
  loop breaker : Memory  Orientation=left
  trailing edge detect : Subsystem
      mask Display: disp('Trailing\nEdge Det')
  outFF : Outport  InitialOutput=0
  wires:
  _timer value (port)/1 -> Relational Operator/2
  1 msec/1 -> Latch1/1(in_1)
  Logical Operator/1 -> Latch1/2(in_2)
  SampHold?1/1(output) -> Sum/2
  Clock/1 -> SampHold?1/1(Input), Sum/1
  Sum/1 -> Relational Operator/1
  Relational Operator/1 -> loop breaker/1, outFF/1
  Latch1/1(out_1) -> SampHold?1/2(S/H?)
  loop breaker/1 -> Logical Operator/3
  Logical Operator1/1 -> Logical Operator/1
  trailing edge detect/1(out_1) -> 1 msec/1, Logical Operator1/1
  Logical Operator2/1 -> Logical Operator/2
  leading edge detect/1(out_1) -> Logical Operator2/1
  event resettable?/1 -> Logical Operator1/2, Logical Operator2/2
  RetFB EnCntrl/1 -> trailing edge detect/1(in_1), leading edge detect/1(in_1)

== system OMSv1_1_SSI/OMSv1.1_SSI 01/27/03/IM CN-LMLN/Saccade Enable/Ret FB sample/event timer4 ==
  note: Resettable
      | Event Timer
  note: (Init input: 0)
  note: (FF init state: Q=0)
  note: (Init input: 0)
  note: In 2) Subsequent events DO NOT reset the counter; it only resets when it
      | reaches zero
  note: 2) A new event (leading or trailing edge) is detected. -- Only case 1)
  note: 1) The count reaches its limit (set in "timer value") -- Both case 1) and 2)
  note: In 1), A leading or trailing edge will reset the counter so that it
      | counts down from the end trailing edge) of that event.
  note: It has TWO modes: 1) Event resettable and 2) Event Non-resettable
  note: The real trick here is understanding how to reload the countdown.
      | It resets if either of two conditions is met:
  note: The "OR" gate allows either of these conditions to reset the circuit.  The delay before the
      | "S" input of the flip-flop prevents both "S" and "R" from being set simultaneously, because
      | this would put the flip-flop in an undefined state.
  note: Therefore, an event first RESETS and then SETS the flip-flop.
  note: This block is an RESETTABLE EVENT TIMER.  It outputs a spike of unit height xx milliseconds
      | (set by "timer value") after it detects an event ( i.e a TRAILING edge which represents the end of a
      |  saccadic pulse)
  RetFB EnCntrl : Inport
  _timer value (port) : Inport  Port=2
  1 msec : TransportDelay  DelayTime=.001
  Clock : Clock
      settings: Decimation=10
  Latch1 : Subsystem  mask(Latch){@1=0}
      mask prompts: @1 "Initial State for Output "Q":"
      mask help: Latch
      mask init:
      | ini=(@1~=0);
      mask Help: Latches the S input.  When S (set) is one, the Q output  becomes one.  The output remains one until the R (reset) input becomes one, forcing the output to zero.  If both R and S are one, the latch will be in an undefined state.
      mask Display: disp('S   Q\n\nR  !Q')
  Logical Operator : Logic  Operator=OR  Inputs=3
  Logical Operator1 : Logic
  Logical Operator2 : Logic
  Relational Operator : RelationalOperator  InputSameDT=on
  SampHold?1 : Subsystem
      mask Display: disp('S&H\n(S=L)\n(H=H)')
  Sum : Sum  Inputs=+-  SaturateOnIntegerOverflow=on  InputSameDT=on
  event resettable? : Constant  Orientation=up  Value=2
  leading edge detect : Subsystem
      mask Display: disp('Leading\nEdge Det')
  loop breaker : Memory  Orientation=left
  trailing edge detect : Subsystem
      mask Display: disp('Trailing\nEdge Det')
  outFF : Outport  InitialOutput=0
  wires:
  RetFB EnCntrl/1 -> trailing edge detect/1(in_1), leading edge detect/1(in_1)
  event resettable?/1 -> Logical Operator1/2, Logical Operator2/2
  leading edge detect/1(out_1) -> Logical Operator2/1
  Logical Operator2/1 -> Logical Operator/2
  trailing edge detect/1(out_1) -> 1 msec/1, Logical Operator1/1
  Logical Operator1/1 -> Logical Operator/1
  loop breaker/1 -> Logical Operator/3
  Latch1/1(out_1) -> SampHold?1/2(S/H?)
  Sum/1 -> Relational Operator/1
  Clock/1 -> SampHold?1/1(Input), Sum/1
  Relational Operator/1 -> outFF/1, loop breaker/1
  SampHold?1/1(output) -> Sum/2
  Logical Operator/1 -> Latch1/2(in_2)
  1 msec/1 -> Latch1/1(in_1)
  _timer value (port)/1 -> Relational Operator/2

== system OMSv1_1_SSI/OMSv1.1_SSI 01/27/03/IM CN-LMLN/Saccade Enable/Ret FB sample/leading edge detect2 ==
  note: It is also possible to remove the SIGNUM function
      | and the '==', and replace them with a simple
      | switch with a threshold of (say) 150 or so.
  note: leading edge detection
  in_1 : Inport
  Abs : Abs  SaturateOnIntegerOverflow=on
  Derivative : Derivative
  Relational Operator : RelationalOperator  Operator===  InputSameDT=on
  Sign : Subsystem
      mask Type: Sign
      mask Description: y = sign(x)
      mask Help: Sign Function:\n\t\t\ty = 1 if x > 0\n\t\t\ty = 0 if x = 0\n\t\t\ty = -1 if x < 0
      mask Display: plot(-50,-50,50,50,[-50,50],[0,0],[0,0],[-50,50],[-40,0],[-30,-30],[0,40],[30,30])
  Threshold 1 : Constant
  out_1 : Outport  InitialOutput=0
  wires:
  Abs/1 -> Derivative/1
  Derivative/1 -> Sign/1(in_1)
  Sign/1(out_1) -> Relational Operator/1
  Threshold 1/1 -> Relational Operator/2
  Relational Operator/1 -> out_1/1
  in_1/1 -> Abs/1

== system OMSv1_1_SSI/OMSv1.1_SSI 01/27/03/IM CN-LMLN/Saccade Enable/Ret FB sample/leading edge detect3 ==
  note: leading edge detection
  note: It is also possible to remove the SIGNUM function
      | and the '==', and replace them with a simple
      | switch with a threshold of (say) 150 or so.
  in_1 : Inport
  Abs : Abs  SaturateOnIntegerOverflow=on
  Derivative : Derivative
  Relational Operator : RelationalOperator  Operator===  InputSameDT=on
  Sign : Subsystem
      mask Type: Sign
      mask Description: y = sign(x)
      mask Help: Sign Function:\n\t\t\ty = 1 if x > 0\n\t\t\ty = 0 if x = 0\n\t\t\ty = -1 if x < 0
      mask Display: plot(-50,-50,50,50,[-50,50],[0,0],[0,0],[-50,50],[-40,0],[-30,-30],[0,40],[30,30])
  Threshold 1 : Constant
  out_1 : Outport  InitialOutput=0
  wires:
  in_1/1 -> Abs/1
  Relational Operator/1 -> out_1/1
  Threshold 1/1 -> Relational Operator/2
  Sign/1(out_1) -> Relational Operator/1
  Derivative/1 -> Sign/1(in_1)
  Abs/1 -> Derivative/1

== system OMSv1_1_SSI/OMSv1.1_SSI 01/27/03/IM CN-LMLN/Saccade Enable/Ret FB sample/leading edge detect4 ==
  note: It is also possible to remove the SIGNUM function
      | and the '==', and replace them with a simple
      | switch with a threshold of (say) 150 or so.
  note: leading edge detection
  in_1 : Inport
  Abs : Abs  SaturateOnIntegerOverflow=on
  Derivative : Derivative
  Relational Operator : RelationalOperator  Operator===  InputSameDT=on
  Sign : Subsystem
      mask Type: Sign
      mask Description: y = sign(x)
      mask Help: Sign Function:\n\t\t\ty = 1 if x > 0\n\t\t\ty = 0 if x = 0\n\t\t\ty = -1 if x < 0
      mask Display: plot(-50,-50,50,50,[-50,50],[0,0],[0,0],[-50,50],[-40,0],[-30,-30],[0,40],[30,30])
  Threshold 1 : Constant
  out_1 : Outport  InitialOutput=0
  wires:
  Abs/1 -> Derivative/1
  Derivative/1 -> Sign/1(in_1)
  Sign/1(out_1) -> Relational Operator/1
  Threshold 1/1 -> Relational Operator/2
  Relational Operator/1 -> out_1/1
  in_1/1 -> Abs/1

== system OMSv1_1_SSI/OMSv1.1_SSI 01/27/03/IM CN-LMLN/Saccade Enable/leading edge detect2/Sign ==
  in_1 : Inport
  Constant : Constant  Value=0
  Relational Operator : RelationalOperator  Operator=>  InputSameDT=on
  Relational Operator1 : RelationalOperator  Operator=<  InputSameDT=on
  Sum : Sum  Inputs=+-  SaturateOnIntegerOverflow=on  InputSameDT=on
  out_1 : Outport  InitialOutput=0
  wires:
  in_1/1 -> Relational Operator/1, Relational Operator1/1
  Constant/1 -> Relational Operator1/2, Relational Operator/2
  Relational Operator1/1 -> Sum/2
  Relational Operator/1 -> Sum/1
  Sum/1 -> out_1/1

== system OMSv1_1_SSI/OMSv1.1_SSI 01/27/03/IM CN-LMLN/Saccade Enable/prolong/Latch1 ==
  in_1 : Inport
  in_2 : Inport  Port=2
  Demux : Demux  Outputs=2
  Logic : CombinatorialLogic  TruthTable=[0 1;0 1;1 0;0 1;1 0;0 1;1 0;1 0]
  Memory : Memory  Orientation=left  X0=ini
  Mux : Mux  Inputs=3
  out_1 : Outport  InitialOutput=0
  out_2 : Outport  Port=2  InitialOutput=0
  wires:
  Demux/2 -> out_2/1
  Logic/1 -> Demux/1
  Mux/1 -> Logic/1
  Demux/1 -> out_1/1, Memory/1
  Memory/1 -> Mux/1
  in_1/1 -> Mux/2
  in_2/1 -> Mux/3

== system OMSv1_1_SSI/OMSv1.1_SSI 01/27/03/IM CN-LMLN/Saccade Enable/prolong/SampHold?2 ==
  note: When "S/H?" is LOW, then "Input" is switched directly to the
      | output ("sample").  When "S/H?" is HIGH, the current output is
      | maintained ("hold").
  Input : Inport
  S/H? : Inport  Port=2
  Memory : Memory  Orientation=left
  Sign : Subsystem
      mask Type: Sign
      mask Description: y = sign(x)
      mask Help: Sign Function:\n\t\t\ty = 1 if x > 0\n\t\t\ty = 0 if x = 0\n\t\t\ty = -1 if x < 0
      mask Display: plot(-50,-50,50,50,[-50,50],[0,0],[0,0],[-50,50],[-40,0],[-30,-30],[0,40],[30,30])
  Switch2 : Switch  Threshold=0.5  SaturateOnIntegerOverflow=on  InputSameDT=on
  output : Outport  InitialOutput=0
  wires:
  Memory/1 -> Switch2/1
  Switch2/1 -> output/1, Memory/1
  Input/1 -> Switch2/3
  Sign/1(out_1) -> Switch2/2
  S/H?/1 -> Sign/1(in_1)

== system OMSv1_1_SSI/OMSv1.1_SSI 01/27/03/IM CN-LMLN/Saccade Enable/prolong/leading edge detect ==
  note: leading edge detection
  in_1 : Inport
  Abs : Abs  SaturateOnIntegerOverflow=on
  Derivative : Derivative
  Relational Operator : RelationalOperator  Operator===  InputSameDT=on
  Sign : Subsystem
      mask Type: Sign
      mask Description: y = sign(x)
      mask Help: Sign Function:\n\t\t\ty = 1 if x > 0\n\t\t\ty = 0 if x = 0\n\t\t\ty = -1 if x < 0
      mask Display: plot(-50,-50,50,50,[-50,50],[0,0],[0,0],[-50,50],[-40,0],[-30,-30],[0,40],[30,30])
  Threshold 1 : Constant
  out_1 : Outport  InitialOutput=0
  wires:
  Abs/1 -> Derivative/1
  Derivative/1 -> Sign/1(in_1)
  Sign/1(out_1) -> Relational Operator/1
  Threshold 1/1 -> Relational Operator/2
  Relational Operator/1 -> out_1/1
  in_1/1 -> Abs/1

== system OMSv1_1_SSI/OMSv1.1_SSI 01/27/03/IM CN-LMLN/Saccade Enable/prolong/trailing edge detect ==
  note: trailing edge detection
  note: It is also possible to remove the SIGNUM function
      | and the '==', and replace them with a simple
      | switch with a threshold of (say) 150 or so.
  in_1 : Inport
  Abs : Abs  SaturateOnIntegerOverflow=on
  Derivative : Derivative
  Relational Operator : RelationalOperator  Operator===  InputSameDT=on
  Sign : Subsystem
      mask Type: Sign
      mask Description: y = sign(x)
      mask Help: Sign Function:\n\t\t\ty = 1 if x > 0\n\t\t\ty = 0 if x = 0\n\t\t\ty = -1 if x < 0
      mask Display: plot(-50,-50,50,50,[-50,50],[0,0],[0,0],[-50,50],[-40,0],[-30,-30],[0,40],[30,30])
  Threshold 1 : Constant  Value=-1
  out_1 : Outport  InitialOutput=0
  wires:
  in_1/1 -> Abs/1
  Relational Operator/1 -> out_1/1
  Threshold 1/1 -> Relational Operator/2
  Sign/1(out_1) -> Relational Operator/1
  Derivative/1 -> Sign/1(in_1)
  Abs/1 -> Derivative/1

== system OMSv1_1_SSI/OMSv1.1_SSI 01/27/03/IM CN-LMLN/Saccade Enable/trailing edge detect/Sign ==
  in_1 : Inport
  Constant : Constant  Value=0
  Relational Operator : RelationalOperator  Operator=>  InputSameDT=on
  Relational Operator1 : RelationalOperator  Operator=<  InputSameDT=on
  Sum : Sum  Inputs=+-  SaturateOnIntegerOverflow=on  InputSameDT=on
  out_1 : Outport  InitialOutput=0
  wires:
  Sum/1 -> out_1/1
  Relational Operator/1 -> Sum/1
  Relational Operator1/1 -> Sum/2
  Constant/1 -> Relational Operator/2, Relational Operator1/2
  in_1/1 -> Relational Operator1/1, Relational Operator/1

== system OMSv1_1_SSI/OMSv1.1_SSI 01/27/03/IM CN-LMLN/Saccade Motor Commmand/TCHNG Override/Latch1 ==
  in_1 : Inport
  in_2 : Inport  Port=2
  Demux : Demux  Outputs=2
  Logic : CombinatorialLogic  TruthTable=[0 1;0 1;1 0;0 1;1 0;0 1;1 0;1 0]
  Memory : Memory  Orientation=left  X0=ini
  Mux : Mux  Inputs=3
  out_1 : Outport  InitialOutput=0
  out_2 : Outport  Port=2  InitialOutput=0
  wires:
  in_2/1 -> Mux/3
  in_1/1 -> Mux/2
  Memory/1 -> Mux/1
  Demux/1 -> Memory/1, out_1/1
  Mux/1 -> Logic/1
  Logic/1 -> Demux/1
  Demux/2 -> out_2/1

== system OMSv1_1_SSI/OMSv1.1_SSI 01/27/03/IM CN-LMLN/Saccade Motor Commmand/TCHNG Override/event timer2 ==
  note: In 2) Subsequent events DO NOT reset the counter; it only resets when it
      | reaches zero
  note: 2) A new event (leading or trailing edge) is detected. -- Only case 1)
  note: 1) The count reaches its limit (set in "timer value") -- Both case 1) and 2)
  note: In 1), Any event (leading or trailing edge) will reset the counter so that it
      | counts down from the end trailing edge) of that event.
  note: It has TWO modes: 1) Event resettable and 2) Event Non-resettable
  note: The real trick here is understanding how to reload the countdown.
      | It resets if either of two conditions is met:
  note: The "OR" gate allows either of these conditions to reset the circuit.  The delay before the
      | "S" input of the flip-flop prevents both "S" and "R" from being set simultaneously, because
      | this would put the flip-flop in an undefined state.
  note: Therefore, an event first RESETS and then SETS the flip-flop.
  note: (Init input: 0)
  note: (FF init state: Q=0)
  note: (Init input: 0)
  note: This block is an RESETTABLE EVENT TIMER.  It outputs a spike of unit height xx milliseconds
      | (set by "timer value") after it detects an event ( i.e a TRAILING edge which represents the end of a
      |  saccadic pulse)
  note: Resettable
      | Event Timer
  _PG : Inport
  _timer value (port) : Inport  Port=2
  1 msec : TransportDelay  DelayTime=.001
  Clock : Clock
      settings: Decimation=10
  Latch1 : Subsystem  mask(Latch){@1=0}
      mask prompts: @1 "Initial State for Output "Q":"
      mask help: Latch
      mask init:
      | ini=(@1~=0);
      mask Help: Latches the S input.  When S (set) is one, the Q output  becomes one.  The output remains one until the R (reset) input becomes one, forcing the output to zero.  If both R and S are one, the latch will be in an undefined state.
      mask Display: disp('S   Q\n\nR  !Q')
  Logical Operator : Logic  Operator=OR  Inputs=3
  Logical Operator1 : Logic
  Logical Operator2 : Logic
  Relational Operator : RelationalOperator  InputSameDT=on
  SampHold?1 : Subsystem
      mask Display: disp('S&H\n(S=L)\n(H=H)')
  Sum : Sum  Inputs=+-  SaturateOnIntegerOverflow=on  InputSameDT=on
  event resettable? : Constant  Orientation=up  Value=0
  leading edge detect : Subsystem
      mask Display: disp('Leading\nEdge Det')
  loop breaker : Memory  Orientation=left
  trailing edge detect : Subsystem
      mask Display: disp('Trailing\nEdge Det')
  out_1 : Outport  InitialOutput=0
  wires:
  event resettable?/1 -> Logical Operator2/2, Logical Operator1/2
  leading edge detect/1(out_1) -> Logical Operator2/1
  Logical Operator2/1 -> Logical Operator/2
  trailing edge detect/1(out_1) -> Logical Operator1/1, 1 msec/1
  Logical Operator1/1 -> Logical Operator/1
  loop breaker/1 -> Logical Operator/3
  _PG/1 -> leading edge detect/1(in_1), trailing edge detect/1(in_1)
  Latch1/1(out_1) -> SampHold?1/2(S/H?)
  Relational Operator/1 -> out_1/1, loop breaker/1
  Sum/1 -> Relational Operator/1
  Clock/1 -> Sum/1, SampHold?1/1(Input)
  SampHold?1/1(output) -> Sum/2
  Logical Operator/1 -> Latch1/2(in_2)
  1 msec/1 -> Latch1/1(in_1)
  _timer value (port)/1 -> Relational Operator/2

== system OMSv1_1_SSI/OMSv1.1_SSI 01/27/03/IM CN-LMLN/Saccade Motor Commmand/TCHNG Override/leading edge detect ==
  note: leading edge detection
  in_1 : Inport
  Abs : Abs  SaturateOnIntegerOverflow=on
  Derivative : Derivative
  Relational Operator : RelationalOperator  Operator===  InputSameDT=on
  Sign : Subsystem
      mask Type: Sign
      mask Description: y = sign(x)
      mask Help: Sign Function:\n\t\t\ty = 1 if x > 0\n\t\t\ty = 0 if x = 0\n\t\t\ty = -1 if x < 0
      mask Display: plot(-50,-50,50,50,[-50,50],[0,0],[0,0],[-50,50],[-40,0],[-30,-30],[0,40],[30,30])
  Threshold 1 : Constant
  out_1 : Outport  InitialOutput=0
  wires:
  in_1/1 -> Abs/1
  Relational Operator/1 -> out_1/1
  Threshold 1/1 -> Relational Operator/2
  Sign/1(out_1) -> Relational Operator/1
  Derivative/1 -> Sign/1(in_1)
  Abs/1 -> Derivative/1

== system OMSv1_1_SSI/OMSv1.1_SSI 01/27/03/IM CN-LMLN/Sampled Target Reconstruction/Boolify/direction1 ==
  in_1 : Inport
  Constant : Constant  Value=0
  Relational Operator : RelationalOperator  Operator=>  InputSameDT=on
  Relational Operator1 : RelationalOperator  Operator=<  InputSameDT=on
  Sum : Sum  Inputs=+-  SaturateOnIntegerOverflow=on  InputSameDT=on
  out_1 : Outport  InitialOutput=0
  wires:
  Sum/1 -> out_1/1
  Relational Operator/1 -> Sum/1
  Relational Operator1/1 -> Sum/2
  Constant/1 -> Relational Operator/2, Relational Operator1/2
  in_1/1 -> Relational Operator1/1, Relational Operator/1

== system OMSv1_1_SSI/OMSv1.1_SSI 01/27/03/IM CN-LMLN/Sampled Target Reconstruction/Boolify1/direction1 ==
  in_1 : Inport
  Constant : Constant  Value=0
  Relational Operator : RelationalOperator  Operator=>  InputSameDT=on
  Relational Operator1 : RelationalOperator  Operator=<  InputSameDT=on
  Sum : Sum  Inputs=+-  SaturateOnIntegerOverflow=on  InputSameDT=on
  out_1 : Outport  InitialOutput=0
  wires:
  in_1/1 -> Relational Operator/1, Relational Operator1/1
  Constant/1 -> Relational Operator1/2, Relational Operator/2
  Relational Operator1/1 -> Sum/2
  Relational Operator/1 -> Sum/1
  Sum/1 -> out_1/1

== system OMSv1_1_SSI/OMSv1.1_SSI 01/27/03/IM CN-LMLN/Sampled Target Reconstruction/Boolify2/direction1 ==
  in_1 : Inport
  Constant : Constant  Value=0
  Relational Operator : RelationalOperator  Operator=>  InputSameDT=on
  Relational Operator1 : RelationalOperator  Operator=<  InputSameDT=on
  Sum : Sum  Inputs=+-  SaturateOnIntegerOverflow=on  InputSameDT=on
  out_1 : Outport  InitialOutput=0
  wires:
  in_1/1 -> Relational Operator/1, Relational Operator1/1
  Constant/1 -> Relational Operator1/2, Relational Operator/2
  Relational Operator1/1 -> Sum/2
  Relational Operator/1 -> Sum/1
  Sum/1 -> out_1/1

== system OMSv1_1_SSI/OMSv1.1_SSI 01/27/03/IM CN-LMLN/Sampled Target Reconstruction/Boolify3/direction1 ==
  in_1 : Inport
  Constant : Constant  Value=0
  Relational Operator : RelationalOperator  Operator=>  InputSameDT=on
  Relational Operator1 : RelationalOperator  Operator=<  InputSameDT=on
  Sum : Sum  Inputs=+-  SaturateOnIntegerOverflow=on  InputSameDT=on
  out_1 : Outport  InitialOutput=0
  wires:
  in_1/1 -> Relational Operator/1, Relational Operator1/1
  Constant/1 -> Relational Operator1/2, Relational Operator/2
  Relational Operator1/1 -> Sum/2
  Relational Operator/1 -> Sum/1
  Sum/1 -> out_1/1
